simulink model "temperature"  (R2019b)
settings: Solver=VariableStepAuto  StartTime=0.0  StopTime=10.0  RelTol=1e-3
settings Model: Creator=jilin  LastModifiedBy=jilin

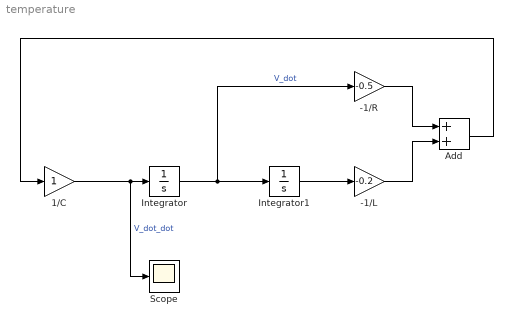
== system temperature ==
  -1/L : Gain  Gain=-0.2
  -1/R : Gain  Gain=-0.5
  1/C : Gain
  Add : Sum
  Integrator : Integrator  InitialCondition=30
  Integrator1 : Integrator
  Scope : Scope
  wires:
  Integrator/1 -> -1/R/1, Integrator1/1  "V_dot"
  1/C/1 -> Scope/1, Integrator/1  "V_dot_dot"
  Integrator1/1 -> -1/L/1
  -1/R/1 -> Add/1
  -1/L/1 -> Add/2
  Add/1 -> 1/C/1
